simulink model "system_model_1"  (R2019a)
settings: Solver=VariableStepAuto  StartTime=0.0  StopTime=50  RelTol=1e-3
values from neighbouring files (symbols this model uses):
  alpha = x(1)    [cost.m]    (also in init.m = 0.6264)
  beta = x(2)    [cost.m]    (also in init.m = 0.9855)
  Kde = x(3)    [cost.m]    (also in init.m = 0.0519)
  Ke = x(4)    [cost.m]    (also in init.m = 0.2421)
undefined symbols (not defined in the file or in its folder): DiscIntNeverNeededParam
libraries: simulink x1
settings Model: Creator=Furka  LastModifiedBy=Furka

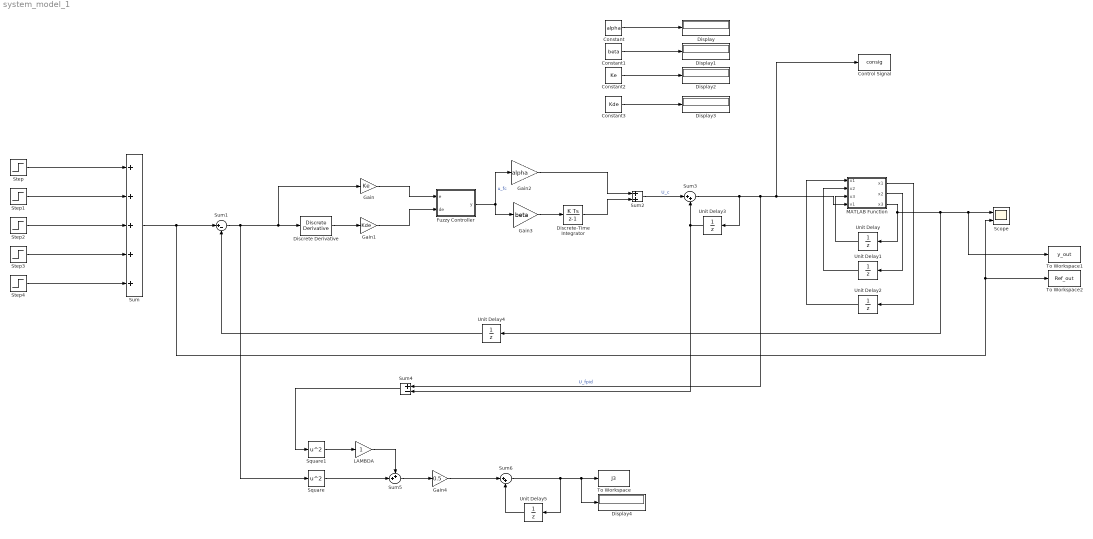
== system system_model_1 ==
  Constant : Constant  Value=alpha
  Constant1 : Constant  Value=beta
  Constant2 : Constant  Value=Ke
  Constant3 : Constant  Value=Kde
  "Control Signal " : ToWorkspace  VariableName=consig  SampleTime=-1
  Discrete Derivative : simulink/Discrete/Discrete Derivative  gainval=1  ICPrevScaledInput=0.0  OutMin=[]  OutMax=[]  OutDataType=fixdt(1, 16)  OutScaling=2^-10  DoSatur=off
  Discrete-Time Integrator : DiscreteIntegrator  SampleTime=0.001  ICPrevOutput=DiscIntNeverNeededParam  ICPrevScaledInput=DiscIntNeverNeededParam
  Display{,1..4} (5 alike) : Display
  "Fuzzy Controller " : MATLAB Function  TreatAsAtomicUnit=on
  Gain : Gain  Gain=Ke
  Gain1 : Gain  Gain=Kde
  Gain2 : Gain  Gain=alpha
  Gain3 : Gain  Gain=beta
  Gain4 : Gain  Gain=0.5
  LAMBDA : Gain
  MATLAB Function : MATLAB Function  TreatAsAtomicUnit=on
  Scope : Scope  NumInputPorts=2
  Square : Math  Operator=square  SaturateOnIntegerOverflow=on
  Square1 : Math  Operator=square  SaturateOnIntegerOverflow=on
  Step : Step  Time=0  After=0.4  SampleTime=0
  Step1 : Step  Time=10  After=0.1  SampleTime=0
  Step2 : Step  Time=20  After=0.1  SampleTime=0
  Step3 : Step  Time=30  After=-0.1  SampleTime=0
  Step4 : Step  Time=40  After=-0.1  SampleTime=0
  Sum : Sum  Inputs=5
  Sum1 : Sum  Inputs=|+-
  Sum2 : Sum
  Sum3 : Sum  Inputs=|++
  Sum4 : Sum  Inputs=+-
  Sum5 : Sum  Inputs=++|
  Sum6 : Sum  Inputs=|++
  To Workspace : ToWorkspace  VariableName=J3  SampleTime=-1
  To Workspace1 : ToWorkspace  VariableName=y_out  SampleTime=-1
  To Workspace2 : ToWorkspace  VariableName=Ref_out  SampleTime=-1
  Unit Delay{,1..5} (6 alike) : UnitDelay  SampleTime=-1  HasFrameUpgradeWarning=on
  wires:
  Step/1 -> Sum/1
  Step1/1 -> Sum/2
  Step2/1 -> Sum/3
  Step3/1 -> Sum/4
  Step4/1 -> Sum/5
  Unit Delay/1 -> MATLAB Function/3("x3 ")
  MATLAB Function/2(x2) -> Unit Delay1/1
  MATLAB Function/1(x1) -> Unit Delay2/1
  Unit Delay1/1 -> MATLAB Function/2("x2 ")
  Unit Delay2/1 -> MATLAB Function/1("x1 ")
  Sum/1 -> Scope/2, To Workspace2/1, Sum1/1
  MATLAB Function/3(x3) -> To Workspace1/1, Scope/1, Unit Delay4/1, Unit Delay/1
  Sum1/1 -> Square/1, Discrete Derivative/1, Gain/1
  "Fuzzy Controller "/1(y) -> Gain2/1, Gain3/1  "u_fc"
  Gain/1 -> "Fuzzy Controller "/1(e)
  Gain1/1 -> "Fuzzy Controller "/2(de)
  Gain2/1 -> Sum2/1
  Sum2/1 -> Sum3/1  "U_c"
  Sum3/1 -> Unit Delay3/1, Sum4/1, "Control Signal "/1, MATLAB Function/4(v1)  "U_fpid"
  Discrete Derivative/1 -> Gain1/1
  Gain3/1 -> Discrete-Time Integrator/1
  Discrete-Time Integrator/1 -> Sum2/2
  Unit Delay3/1 -> Sum4/2, Sum3/2
  Unit Delay4/1 -> Sum1/2
  Sum4/1 -> Square1/1
  Square/1 -> Sum5/2
  Sum5/1 -> Gain4/1
  Gain4/1 -> Sum6/1
  Sum6/1 -> Unit Delay5/1, Display4/1, To Workspace/1
  Unit Delay5/1 -> Sum6/2
  Constant/1 -> Display/1
  Constant1/1 -> Display1/1
  Constant2/1 -> Display2/1
  Constant3/1 -> Display3/1
  LAMBDA/1 -> Sum5/1
  Square1/1 -> LAMBDA/1

== matlab function system_model_1/Fuzzy Controller  ==
  data: e input; y output; de input
function y = fcn(e,de)
    e_2 = -1;
    e_1 = -0.4;
    e0 = 0;
    e1 = 0.4;
    e2 = 1;
    
    %fuzzification
    A_1 = (e0 - e) / (e0 - e_1);
    A_2 = (e_1 - e) / (e_1 - e_2);
    A0 = (e1 - e) / (e1 - e0);
    A1 = (e - e0) / (e1 - e0);
    A2 = (e - e1) / (e2 - e1);

    B_1 = (e0 - de) / (e0 - e_1);
    B_2 = (e_1 - de) / (e_1 - e_2);
    B0 = (e1 - de) / (e1 - e0);  
    B1 = (de - e0) / (e1 - e0);
    B2 = (de - e1) / (e2 - e1);
    
    u_fc = 0;
    
    if(e_2 <= e && e <= e_1)
        
        if(e_2 <= de && de <= e_1)
            u_11 = -1;
            u_21 = -0.7;
            u_12 = -0.7;
            u_22 = -0.4;
            u_fc = ((A_2*B_2*u_11)+(A_1*B_2*u_21)+(A_2*B_1*u_12)+(A_1*B_1*u_22));
            
        elseif(e_1 <= de && de <= e0)
            u_11 = -0.7;
            u_21 = -0.4;
            u_12 = -0.5;
            u_22 = -0.2;
            u_fc = ((A_2*B_1*u_11)+(A_1*B_1*u_21)+(A_2*B0*u_12)+(A_1*B0*u_22));   

        elseif(e0 <= de && de <= e1)
            u_11 = -0.5;
            u_21 = -0.2;
            u_12 = -0.3;
            u_22 = 0;
            u_fc = ((A_2*B0*u_11)+(A_1*B0*u_21)+(A_2*B1*u_12)+(A_1*B1*u_22));
            
        elseif(e1 <= de && de <= e2)
            u_11 = -0.3;
            u_21 = 0;
            u_12 = 0;
            u_22 = 0.3;
            u_fc = ((A_2*B1*u_11)+(A_1*B1*u_21)+(A_2*B2*u_12)+(A_1*B2*u_22));
            
        end
        
    end

    if(e_1 <= e && e <= e0)
        
        if(e_2 <= de && de <= e_1)
            u_11 = -0.7;
            u_21 = -0.5;
            u_12 = -0.4;
            u_22 = -0.2;
            u_fc = ((A_1*B_2*u_11)+(A0*B_2*u_21)+(A_1*B_1*u_12)+(A0*B_1*u_22));
            
        elseif(e_1 <= de && de <= e0)
            u_11 = -0.4;
            u_21 = -0.2;
            u_12 = -0.2;
            u_22 = 0;
            u_fc = ((A_1*B_1*u_11)+(A0*B_1*u_21)+(A_1*B0*u_12)+(A0*B0*u_22));
            
        elseif(e0 <= de && de <= e1)
            u_11 = -0.2;
            u_21 = 0;
            u_12 = 0;
            u_22 = 0.2;
            u_fc = ((A_1*B0*u_11)+(A0*B0*u_21)+(A_1*B1*u_12)+(A0*B1*u_22));
            
        elseif(e1 <= de && de <= e2)
            u_11 = 0;
            u_21 = 0.2;
            u_12 = 0.3;
            u_22 = 0.5;
            u_fc = ((A_1*B1*u_11)+(A0*B1*u_21)+(A_1*B2*u_12)+(A0*B2*u_22));
            
        end
        
    end

    if(e0 <= e && e <= e1)
        
        if(e_2 <= de && de <= e_1)
            u_11 = -0.5;
            u_21 = -0.3;
            u_12 = -0.2;
            u_22 = 0;
            u_fc = ((A0*B_2*u_11)+(A1*B_2*u_21)+(A0*B_1*u_12)+(A1*B_1*u_22));
            
        elseif(e_1 <= de && de <= e0)
            u_11 = -0.2;
            u_21 = 0;
            u_12 = 0;
            u_22 = 0.2;
            u_fc = ((A0*B_1*u_11)+(A1*B_1*u_21)+(A0*B0*u_12)+(A1*B0*u_22));
            
        elseif(e0 <= de && de <= e1)
            u_11 = 0;
            u_21 = 0.2;
            u_12 = 0.2;
            u_22 = 0.4;
            u_fc = ((A0*B0*u_11)+(A1*B0*u_21)+(A0*B1*u_12)+(A1*B1*u_22));
            
        elseif(e1 <= de && de <= e2)
            u_11 = 0.2;
            u_21 = 0.4;
            u_12 = 0.5;
            u_22 = 0.7;
            u_fc = ((A0*B1*u_11)+(A1*B1*u_21)+(A0*B2*u_12)+(A1*B2*u_22));
            
        end
        
    end

    if(e1 <= e && e <= e2)
        
        if(e_2 <= de && de <= e_1)
            u_11 = -0.3;
            u_21 = 0;
            u_12 = 0;
            u_22 = 0.3;
            u_fc = ((A1*B_2*u_11)+(A2*B_2*u_21)+(A1*B_1*u_12)+(A2*B_1*u_22));
            
        elseif(e_1 <= de && de <= e0)
            u_11 = 0;
            u_21 = 0.3;
            u_12 = 0.2;
            u_22 = 0.5;
            u_fc = ((A1*B_1*u_11)+(A2*B_1*u_21)+(A1*B0*u_12)+(A2*B0*u_22));
            
        elseif(e0 <= de && de <= e1)
            u_11 = 0.2;
            u_21 = 0.5;
            u_12 = 0.4;
            u_22 = 0.7;
            u_fc = ((A1*B0*u_11)+(A2*B0*u_21)+(A1*B1*u_12)+(A2*B1*u_22));
            
        elseif(e1 <= de && de <= e2)
            u_11 = 0.4;
            u_21 = 0.7;
            u_12 = 0.7;
            u_22 = 1;
            u_fc = ((A1*B1*u_11)+(A2*B1*u_21)+(A1*B2*u_12)+(A2*B2*u_22));
            
        end
        
    end

y = u_fc;

== matlab function system_model_1/MATLAB Function ==
  data: x1 input; x1 output; x2 input; x3 input; v1 input; x2 output; x3 output
% function y = fcn(u)
% 
% y = u;

function  [x1,x2,x3]=CSTR_runga_kutta_model(x1,x2,x3,v1)

Da1=3;
Da2=0.5;
Da3=1;
d2=1;
h = 0.01;

k1x1=1-x1-Da1*x1+Da2*x2*x2;
k1x2=-x2+Da1*x1-Da2*x2*x2-Da3*d2*x2*x2+v1;
k1x3=-x3+Da3*d2*x2*x2;



k2x1=1-(x1+h*k1x1/2)-Da1*(x1+h*k1x1/2)+Da2*(x2+h*k1x2/2)*(x2+h*k1x2/2);
k2x2=-(x2+h*k1x2/2)+Da1*(x1+h*k1x1/2)-Da2*(x2+h*k1x2/2)*(x2+h*k1x2/2)-Da3*d2*(x2+h*k1x2/2)*(x2+h*k1x2/2)+v1;
k2x3=-(x3+h*k1x3/2)+Da3*d2*(x2+h*k1x2/2)*(x2+h*k1x2/2);


k3x1=1-(x1+h*k2x1/2)-Da1*(x1+h*k2x1/2)+Da2*(x2+h*k2x2/2)*(x2+h*k2x2/2);
k3x2=-(x2+h*k2x2/2)+Da1*(x1+h*k2x1/2)-Da2*(x2+h*k2x2/2)*(x2+h*k2x2/2)-Da3*d2*(x2+h*k2x2/2)*(x2+h*k2x2/2)+v1;
k3x3=-(x3+h*k2x3/2)+Da3*d2*(x2+h*k2x2/2)*(x2+h*k2x2/2);



k4x1=1-(x1+h*k3x1)-Da1*(x1+h*k3x1)+Da2*(x2+h*k3x2)*(x2+h*k3x2);
k4x2=-(x2+h*k3x2)+Da1*(x1+h*k3x1)-Da2*(x2+h*k3x2)*(x2+h*k3x2)-Da3*d2*(x2+h*k3x2)*(x2+h*k3x2)+v1;
k4x3=-(x3+h*k3x3)+Da3*d2*(x2+h*k3x2)*(x2+h*k3x2);



x1=x1+(h/6)*(k1x1+2*k2x1+2*k3x1+k4x1);
x2=x2+(h/6)*(k1x2+2*k2x2+2*k3x2+k4x2);
x3=x3+(h/6)*(k1x3+2*k2x3+2*k3x3+k4x3);
